simulink model "regenerative_braking_model_prototype_1"  (R2025a)
settings: Solver=ode23tb  StartTime=0.0  StopTime=70  RelTol=1e-3
undefined symbols (not defined in the file or in its folder): Ion, Lithium
libraries: spsMosfetLib x5, spsSeriesRLCBranchLib x4, spsBatteryLib x1, spsCurrentMeasurementLib x1, spsDCMachineLib x1, spsDCVoltageSourceLib x1, spsDiodeLib x1, spsGroundLib x1, SignalEditorBlockLib x1, spsVoltageMeasurementLib x1, sps_lib x1
settings Model: Creator=Shubham  LastModifiedBy=Shubham

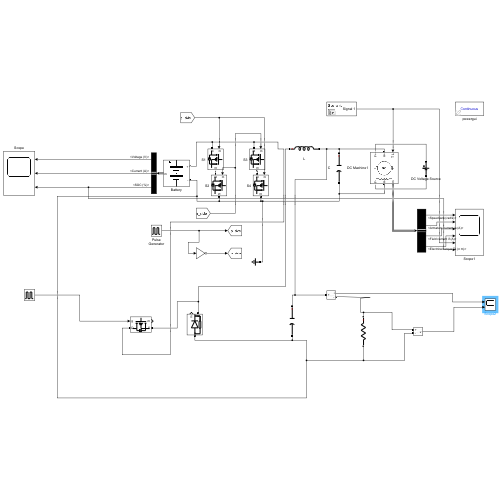
[thumbnail: Simulink's stored preview of the top-level diagram]
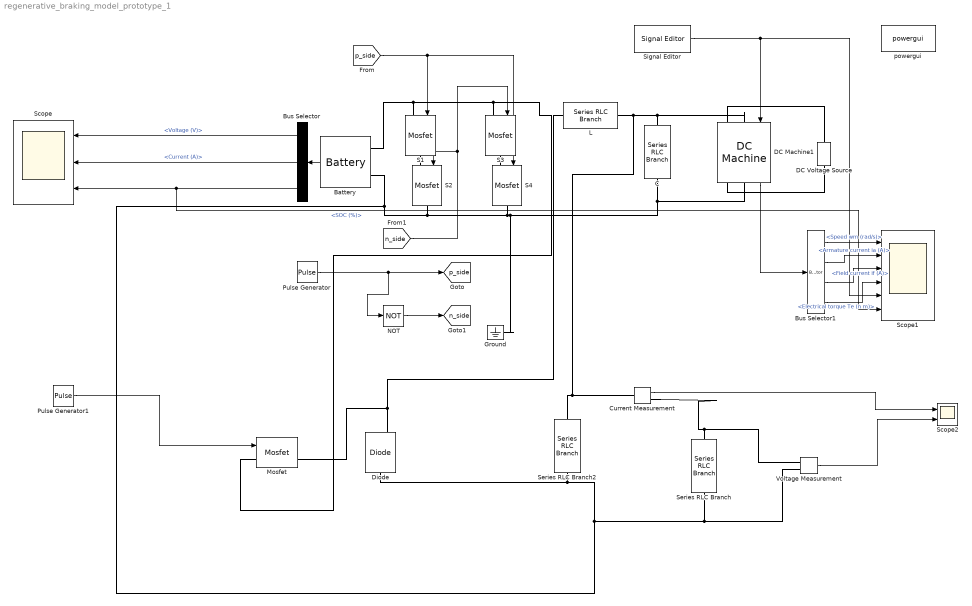
== system regenerative_braking_model_prototype_1 ==
  " S2" : spsMosfetLib/Mosfet  Ron=0.1  Lon=0  Rd=0.01  Vfd=0  IC=0  Rs=1e5  Cs=inf  Measurements=off
  Battery : spsBatteryLib/Battery  BatType=Lithium-Ion  NomV=60  NomQ=20  SOC=90  Batt_Tr=30  PresetModel=on  MaxQ=20  MinV=45  FullV=69.8392  Dis_rate=8.6957  R=0.03  Normal_OP=18.087  expZone="[64.8232     0.982609]"
  Bus Selector : BusSelector  OutputSignals=Voltage (V),Current (A),SOC (%)
  Bus Selector1 : BusSelector  OutputSignals=Speed wm (rad/s),Armature current ia (A),Field current if (A),Electrical torque Te (n m)
  C : spsSeriesRLCBranchLib/Series RLC Branch  LConnTagsString=__new0  RConnTagsString=__new0  BranchType=C  Resistance=1  Inductance=1e-3  SetiL0=off  InitialCurrent=0  Capacitance=470e-6  Setx0=off  InitialVoltage=0  Measurements=None
  Current Measurement : spsCurrentMeasurementLib/Current Measurement  PhasorSimulation=off  OutputType=Complex  PSBequivalent=0
  DC Machine1 : spsDCMachineLib/DC Machine  PresetModel=01: 5HP 240V 1750RPM Field:300V  MechanicalLoad=Torque TL  FieldType=Wound  ShowDetailedParameters=on  MeasurementBus=off  RLa=[2.581 0.028]  RLf=[281.2 156]  Laf=0.9483  MachineConstant=Torque constant (N.m/A)  Ke=1.8  Kt=1.8  J=0.02215  Bm=0.002953  Tf=0.5161  w0=1  Ifinit=1.06685633001422  TsPowergui=0  TsBlock=-1
  DC Voltage Source : spsDCVoltageSourceLib/DC Voltage Source  Amplitude=300  Measurements=None
  Diode : spsDiodeLib/Diode  Ron=0.001  Lon=0  Vf=0.8  IC=0  UseSnubber=0  Rs=500  Cs=250e-9  Measurements=on
  Ground : spsGroundLib/Ground  LConnTagsString=a
  L : spsSeriesRLCBranchLib/Series RLC Branch  LConnTagsString=__new0  RConnTagsString=__new0  BranchType=L  Resistance=1  Inductance=1.5e-3  SetiL0=off  InitialCurrent=0  Capacitance=1e-6  Setx0=off  InitialVoltage=0  Measurements=None
  Mosfet : spsMosfetLib/Mosfet  Ron=0.1  Lon=0  Rd=0.01  Vfd=0  IC=0  Rs=1e5  Cs=inf  Measurements=on
  NOT : Logic  Operator=NOT  IconShape=distinctive  AllPortsSameDT=off  OutDataTypeStr=boolean
  Pulse Generator : DiscretePulseGenerator  PulseType=Time based  Period=50e-6  PulseWidth=25
  Pulse Generator1 : DiscretePulseGenerator  PulseType=Time based  Period=50e-6  PulseWidth=23.3
  S1 : spsMosfetLib/Mosfet  Ron=0.1  Lon=0  Rd=0.01  Vfd=0  IC=0  Rs=1e5  Cs=inf  Measurements=off
  S3 : spsMosfetLib/Mosfet  Ron=0.1  Lon=0  Rd=0.01  Vfd=0  IC=0  Rs=1e5  Cs=inf  Measurements=off
  S4 : spsMosfetLib/Mosfet  Ron=0.1  Lon=0  Rd=0.01  Vfd=0  IC=0  Rs=1e5  Cs=inf  Measurements=off
  Scope : Scope  NumInputPorts=3
      settings: ActiveDisplayYMinimum=69.4711331352431  ActiveDisplayYMaximum=92.882407303165365
  Scope1 : Scope  NumInputPorts=6
      settings: ActiveDisplayYMinimum=-135.91054417370253  ActiveDisplayYMaximum=81.027604972815084
  Scope2 : Scope  NumInputPorts=2
      settings: ActiveDisplayYMinimum=2.8758192411863153  ActiveDisplayYMaximum=33.538412811299168  DataLoggingVariableName=ScopeData2
  Series RLC Branch : spsSeriesRLCBranchLib/Series RLC Branch  LConnTagsString=__new0  RConnTagsString=__new0  BranchType=R  Resistance=46.1  Inductance=1e-3  SetiL0=off  InitialCurrent=0  Capacitance=1e-6  Setx0=off  InitialVoltage=0  Measurements=None
  Series RLC Branch2 : spsSeriesRLCBranchLib/Series RLC Branch  LConnTagsString=__new0  RConnTagsString=__new0  BranchType=C  Resistance=1  Inductance=1e-3  SetiL0=off  InitialCurrent=0  Capacitance=100e-6  Setx0=off  InitialVoltage=0  Measurements=None
  Signal Editor : SignalEditorBlockLib/Signal Editor  FileName=signal builder torque steps.mat  ActiveScenario=Scenario  ActiveSignal=Signal 1  IsBus=off  OutputBusObjectStr=Bus: BusObject  SampleTime=0  ZeroCross=off  OutputAfterFinalValue=Setting to zero  Unit=inherit  PreserveSignalName=on  ApplySigPropsToAllScenarios=on  ApplySigPropsToAllSignals=off  SignalPropertySource=Dialog parameters
  Voltage Measurement : spsVoltageMeasurementLib/Voltage Measurement  PhasorSimulation=off  OutputType=Complex  PSBequivalent=0
  powergui : sps_lib/powergui  Priority=1  SimulationMode=Continuous  SampleTime=50e-6  frequency=60  Iterations=50  frequencyindice=0  Pbase=100e6  ErrMax=1e-4  UnitsV=kV  UnitsW=MW  buscounter=0  FunctionMessages=off  echomessages=off  EnableUseOfTLC=off  CurrentSourceSwitches=off  DisableSnubberDevices=off  DisableRonSwitches=off  DisableVfSwitches=off  DisplayEquations=off  AutomaticDiscreteSolvers=off  SolverType=Tustin/Backward Euler (TBE)  Interpol=off  ExternalGateDelay=off  methode=off  Ts=100  x0status=blocks  SPID=on  SwTol=0  HookPort=off  NonlinearTolerance=1e-4  nMaxIteration=100  ContinueOnMaxIteration=off  RestoreLinks=warning  ResistiveCurrentMeasurement=off  Frange=[0:2:500]  Ylog=off  Xlog=on  ShowGrid=off  save=off  variable=ZData  structure=0  ZoomFFT=off  StartTime=0.0  cycles=1  DisplayStyle=1  fundamental=60  FreqAxis=off  MaxFrequency=1000  frequencyindicesteady=1  RmsSteady=1  display=off
  tag scope: n_side=global, p_side=global
  wires:
  Signal Editor/1 -> Scope1/5, DC Machine1/1
  Battery/1 -> Bus Selector/1
  Bus Selector/1 -> Scope/1  "<Voltage (V)>"
  Bus Selector/2 -> Scope/2  "<Current (A)>"
  Bus Selector/3 -> Scope1/6, Scope/3  "<SOC (%)>"
  DC Machine1/1 -> Bus Selector1/1
  Bus Selector1/2 -> Scope1/2  "<Armature current ia (A)>"
  Bus Selector1/1 -> Scope1/1  "<Speed wm (rad/s)>"
  Bus Selector1/4 -> Scope1/4  "<Electrical torque Te (n m)>"
  Bus Selector1/3 -> Scope1/3  "<Field current if (A)>"
  Pulse Generator/1 -> NOT/1, [p_side]
  NOT/1 -> [n_side]
  [p_side] -> S4/1, S1/1
  [n_side] -> S3/1, " S2"/1
  Pulse Generator1/1 -> Mosfet/1
  Voltage Measurement/1 -> Scope2/2
  Current Measurement/1 -> Scope2/1
  connections:
  DC Voltage Source/RConn1 -- DC Machine1/LConn2
  DC Voltage Source/LConn1 -- DC Machine1/RConn2
  S1/LConn1 -- Battery/LConn1 -- Mosfet/LConn1 -- S3/LConn1
  S3/RConn1 -- S4/LConn1
  S1/RConn1 -- " S2"/LConn1
  Series RLC Branch/LConn1 -- Current Measurement/RConn1 -- Voltage Measurement/LConn1
  L/RConn1 -- Series RLC Branch2/LConn1 -- Current Measurement/LConn1 -- DC Machine1/LConn1 -- C/LConn1
  " S2"/RConn1 -- Series RLC Branch2/RConn1 -- Diode/LConn1 -- Series RLC Branch/RConn1 -- Voltage Measurement/LConn2 -- Battery/LConn2 -- Ground/LConn1 -- DC Machine1/RConn1 -- C/RConn1 -- S4/RConn1
  L/LConn1 -- Diode/RConn1 -- Mosfet/RConn1
